simulink model "ASDrf_Governor"  (R2016b)
settings: configuration reference "CodeGenConfigSet" (kept outside this file)
values from neighbouring files (symbols this model uses):
  ASDrf_KpFltCurr_C = Calibration.Parameter    [init_ASDrf_Governor.m]    (also in init_ASDrf_Governor_SIL.m = Simulink.Parameter)
  ASDrf_swtLim_C = Calibration.Parameter    [init_ASDrf_Governor.m]    (also in init_ASDrf_Governor_SIL.m = Simulink.Parameter)
  ASDrf_swtSpdGovCor_C = Calibration.Parameter    [init_ASDrf_Governor.m]    (also in init_ASDrf_Governor_SIL.m = Simulink.Parameter)
  ASDrf_trqSteepNeg_C = Calibration.Parameter    [init_ASDrf_Governor.m]    (also in init_ASDrf_Governor_SIL.m = Simulink.Parameter)
  ASDrf_trqSteepPos_C = Calibration.Parameter    [init_ASDrf_Governor.m]    (also in init_ASDrf_Governor_SIL.m = Simulink.Parameter)
  ASDrf_trqThresNeg_C = Calibration.Parameter    [init_ASDrf_Governor.m]    (also in init_ASDrf_Governor_SIL.m = Simulink.Parameter)
  ASDrf_trqThresPos_C = Calibration.Parameter    [init_ASDrf_Governor.m]    (also in init_ASDrf_Governor_SIL.m = Simulink.Parameter)
  TRQ_MAX = fi(1000,Trq_Nm)    [init_ASDrf_Governor.m]    (also in init_ASDrf_Governor_SIL.m)
  TRQ_MIN = fi(-3276,Trq_Nm)    [init_ASDrf_Governor.m]    (also in init_ASDrf_Governor_SIL.m)
libraries: simulink x10, CXLib x4
settings Model: Creator=lenovo  LastModifiedBy=lenovo
settings ConfigSetRef: SourceLocation=Base Workspace

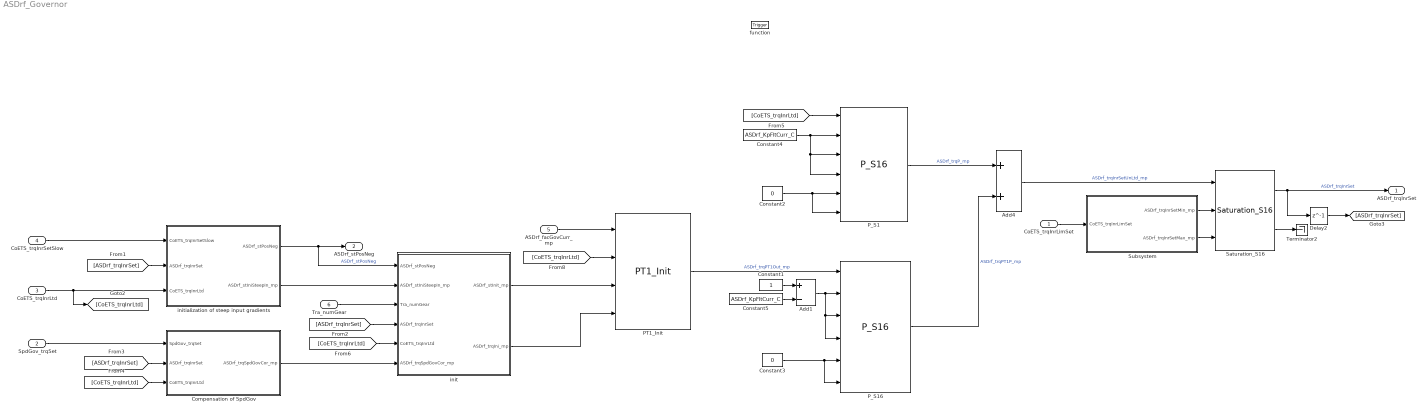
== system ASDrf_Governor ==
  CoETS_trqInrLimSet : Inport  Tag=Nm  Description=Limitation torque without the part of the speed governor  OutMin=-3000  OutMax=3000  OutDataTypeStr=Trq_Nm
  SpdGov_trqSet : Inport  Tag=Nm  Description=Set point torque of SpdGov on the fuel path  Port=2  OutMin=-3000  OutMax=3000  OutDataTypeStr=Trq_Nm
  CoETS_trqInrLtd : Inport  Tag=Nm  Description=inner torque set value after limitation, before AS  Port=3  OutMin=-3000  OutMax=3000  OutDataTypeStr=Trq_Nm
  CoETS_trqInrSetSlow : Inport  Tag=Nm  Description=Filtered inner torque ( positive torque) desired value (standard signal path) generated out of CoPT_trqDesEng  Port=4  OutMin=-3276  OutMax=3276  OutDataTypeStr=Trq_Nm
  ASDrf_facGovCurr_mp : Inport  Description=Active state after priorisation (decimal coded)  Port=5  OutMin=0  OutMax=99.9  OutDataTypeStr=PT_fac
  Tra_numGear : Inport  Description=Current gear information  Port=6  OutMin=-128  OutMax=127  OutDataTypeStr=Tra_num
  function : TriggerPort  TriggerType=function-call  VariantControl=Variant
  Add1 : Sum  Inputs=+-  SaturateOnIntegerOverflow=on  InputSameDT=on
  Add4 : Sum  SaturateOnIntegerOverflow=on  InputSameDT=on
  Compensation of SpdGov : Subsystem
  Constant1 : Constant  RequirementInfo={'other' 'APP_requirements.doc' '@Simulink_requirement_item_25' 'true' '手动开关' '' } %GIDa_04e9130c_3732_46d4_8727_99cf29214165  OutDataTypeStr=Inherit: Inherit via back propagation
  Constant2 : Constant  RequirementInfo={'other' 'APP_requirements.doc' '@Simulink_requirement_item_25' 'true' '手动开关' '' } %GIDa_94a70317_27f7_4a67_bc50_074724e5fa22  Value=0  OutDataTypeStr=Inherit: Inherit via back propagation
  Constant3 : Constant  RequirementInfo={'other' 'APP_requirements.doc' '@Simulink_requirement_item_25' 'true' '手动开关' '' } %GIDa_3fa9db96_13e9_4b77_bcb7_da159fb74a91  Value=0  OutDataTypeStr=Inherit: Inherit via back propagation
  Constant4 : Constant  RequirementInfo={'other' 'APP_requirements.doc' '@Simulink_requirement_item_25' 'true' '手动开关' '' } %GIDa_2e8aa955_92f2_4b22_b779_7d16fefc9cfa  Value=ASDrf_KpFltCurr_C
  Constant5 : Constant  RequirementInfo={'other' 'APP_requirements.doc' '@Simulink_requirement_item_25' 'true' '手动开关' '' } %GIDa_b568d7eb_b45f_4e62_9df6_34760f8c3a7b  Value=ASDrf_KpFltCurr_C
  Delay2 : Delay  DelayLength=1  InitialCondition=0
  PT1_Init : CXLib/PT1_Init
  P_S1 : CXLib/P_S16
  P_S16 : CXLib/P_S16
  Saturation_S16 : CXLib/Saturation_S16
  Subsystem : Subsystem
  Terminator2 : Terminator
  init : Subsystem
  "initialization of steep input gradients " : Subsystem
  ASDrf_trqInrSet : Outport  Tag=Nm  Description=ASD reference filter torque output  OutMin=-3000  OutMax=3000  OutDataTypeStr=Trq_Nm
  ASDrf_stPosNeg : Outport  Description=Positive or negative intervention status  Port=2  OutMin=0  OutMax=1  OutDataTypeStr=boolean
  wires:
  [CoETS_trqInrLtd] -> init/5(CoETS_trqInrLtd)
  Delay2/1 -> [ASDrf_trqInrSet]
  [CoETS_trqInrLtd] -> PT1_Init/2
  Subsystem/2(ASDrf_trqInrSetMax_mp) -> Saturation_S16/3
  Subsystem/1(ASDrf_trqInrSetMin_mp) -> Saturation_S16/2
  CoETS_trqInrLimSet/1 -> Subsystem/1(CoETS_trqInrLimSet)
  "initialization of steep input gradients "/1(ASDrf_stPosNeg) -> ASDrf_stPosNeg/1, init/1(ASDrf_stPosNeg)  "ASDrf_stPosNeg"
  Constant2/1 -> P_S1/6, P_S1/5
  Saturation_S16/2 -> Terminator2/1
  Constant1/1 -> Add1/1
  [ASDrf_trqInrSet] -> Compensation of SpdGov/2(ASDrf_trqInrSet)
  Saturation_S16/1 -> ASDrf_trqInrSet/1, Delay2/1  "ASDrf_trqInrSet"
  P_S16/1 -> Add4/2  "ASDrf_trqPT1P_mp"
  P_S1/1 -> Add4/1  "ASDrf_trqP_mp"
  Constant3/1 -> P_S16/5, P_S16/6
  Add1/1 -> P_S16/2, P_S16/3, P_S16/4
  init/1(ASDrf_stInit_mp) -> PT1_Init/3
  Constant5/1 -> Add1/2
  [ASDrf_trqInrSet] -> init/4(ASDrf_trqInrSet)
  CoETS_trqInrSetSlow/1 -> "initialization of steep input gradients "/1(CoETS_trqInrSetSlow)
  PT1_Init/1 -> P_S16/1  "ASDrf_trqPT1Out_mp"
  [ASDrf_trqInrSet] -> "initialization of steep input gradients "/2(ASDrf_trqInrSet)
  Compensation of SpdGov/1(ASDrf_trqSpdGovCor_mp) -> init/6(ASDrf_trqSpdGovCor_mp)
  init/2(ASDrf_trqIni_mp) -> PT1_Init/4
  Tra_numGear/1 -> init/3(Tra_numGear)
  "initialization of steep input gradients "/2(ASDrf_stIniSteepIn_mp) -> init/2(ASDrf_stIniSteepIn_mp)
  CoETS_trqInrLtd/1 -> [CoETS_trqInrLtd], "initialization of steep input gradients "/3(CoETS_trqInrLtd)
  ASDrf_facGovCurr_mp/1 -> PT1_Init/1
  [CoETS_trqInrLtd] -> Compensation of SpdGov/3(CoETS_trqInrLtd)
  [CoETS_trqInrLtd] -> P_S1/1
  Add4/1 -> Saturation_S16/1  "ASDrf_trqInrSetUnLtd_mp"
  Constant4/1 -> P_S1/2, P_S1/3, P_S1/4
  SpdGov_trqSet/1 -> Compensation of SpdGov/1(SpdGov_trqSet)

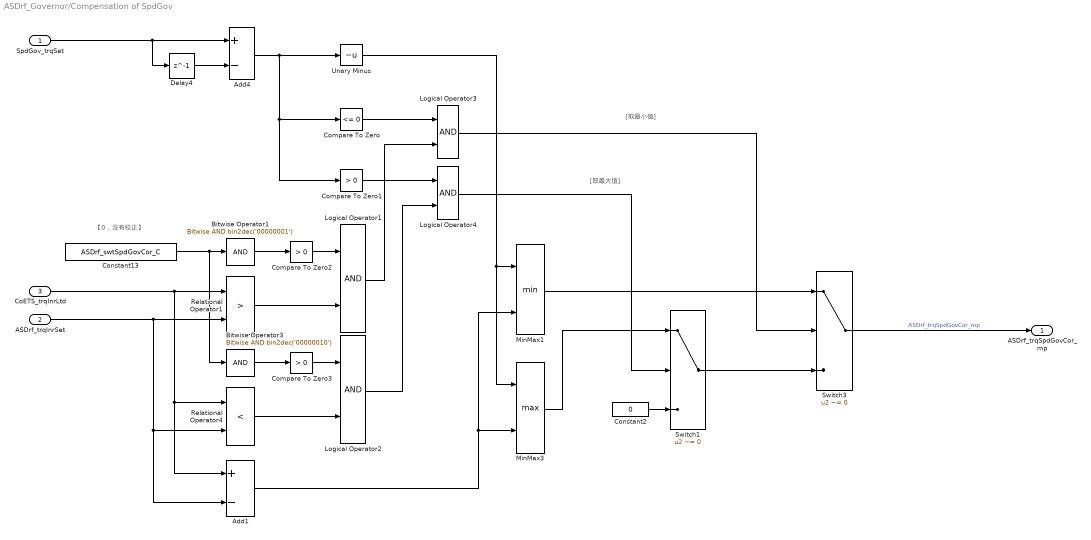
== system ASDrf_Governor/Compensation of SpdGov ==
  note: [取最大值]
  note: [取最小值]
  note: 【0，没有校正】
  SpdGov_trqSet : Inport
  ASDrf_trqInrSet : Inport  Port=2
  CoETS_trqInrLtd : Inport  Port=3
  Add1 : Sum  Inputs=+-  SaturateOnIntegerOverflow=on  InputSameDT=on
  Add4 : Sum  Inputs=+-  SaturateOnIntegerOverflow=on  InputSameDT=on
  Bitwise Operator1 : simulink/Logic and Bit Operations/Bitwise Operator  logicop=AND  UseBitMask=on  BitMask=bin2dec('00000001')  BitMaskRealWorld=Stored Integer
  Bitwise Operator3 : simulink/Logic and Bit Operations/Bitwise Operator  logicop=AND  UseBitMask=on  BitMask=bin2dec('00000010')  BitMaskRealWorld=Stored Integer
  Compare To Zero : simulink/Logic and Bit Operations/Compare To Zero  relop=<=  OutDataTypeStr=boolean
  Compare To Zero1 : simulink/Logic and Bit Operations/Compare To Zero  relop=>  OutDataTypeStr=boolean
  Compare To Zero2 : simulink/Logic and Bit Operations/Compare To Zero  relop=>  OutDataTypeStr=boolean
  Compare To Zero3 : simulink/Logic and Bit Operations/Compare To Zero  relop=>  OutDataTypeStr=boolean
  Constant13 : Constant  RequirementInfo={'other' 'APP_requirements.doc' '@Simulink_requirement_item_25' 'true' '手动开关' '' } %GIDa_336f8dde_0a6f_4504_9b94_889caf0ed8bc  Value=ASDrf_swtSpdGovCor_C  SampleTime=-1
  Constant2 : Constant  RequirementInfo={'other' 'APP_requirements.doc' '@Simulink_requirement_item_25' 'true' '手动开关' '' } %GIDa_e3fc0150_ba4b_4eb3_baf9_a854b361ddb2  Value=0  OutDataTypeStr=Inherit: Inherit via back propagation
  Delay4 : Delay  DelayLength=1  InitialCondition=0
  Logical Operator{1..4} (4 alike) : Logic  OutDataTypeStr=boolean
  MinMax1 : MinMax  Inputs=2  SaturateOnIntegerOverflow=on  InputSameDT=on
  MinMax3 : MinMax  Function=max  Inputs=2  SaturateOnIntegerOverflow=on  InputSameDT=on
  Relational Operator1 : RelationalOperator  Operator=>  OutDataTypeStr=boolean  RndMeth=Simplest  InputSameDT=on
  Relational Operator4 : RelationalOperator  Operator=<  OutDataTypeStr=boolean  RndMeth=Simplest  InputSameDT=on
  Switch1 : Switch  Criteria=u2 ~= 0  SaturateOnIntegerOverflow=on  InputSameDT=on
  Switch3 : Switch  Criteria=u2 ~= 0  SaturateOnIntegerOverflow=on  InputSameDT=on
  Unary Minus : UnaryMinus
  ASDrf_trqSpdGovCor_mp : Outport
  wires:
  Compare To Zero3/1 -> Logical Operator2/1
  Bitwise Operator3/1 -> Compare To Zero3/1
  Compare To Zero2/1 -> Logical Operator1/1
  Constant13/1 -> Bitwise Operator3/1, Bitwise Operator1/1
  SpdGov_trqSet/1 -> Add4/1, Delay4/1
  Switch3/1 -> ASDrf_trqSpdGovCor_mp/1  "ASDrf_trqSpdGovCor_mp"
  Logical Operator1/1 -> Logical Operator3/2
  MinMax1/1 -> Switch3/1
  ASDrf_trqInrSet/1 -> Relational Operator1/2, Relational Operator4/2, Add1/2
  Compare To Zero1/1 -> Logical Operator4/1
  Compare To Zero/1 -> Logical Operator3/1
  CoETS_trqInrLtd/1 -> Relational Operator1/1, Relational Operator4/1, Add1/1
  Relational Operator1/1 -> Logical Operator1/2
  Add4/1 -> Unary Minus/1, Compare To Zero1/1, Compare To Zero/1
  Bitwise Operator1/1 -> Compare To Zero2/1
  MinMax3/1 -> Switch1/1
  Relational Operator4/1 -> Logical Operator2/2
  Logical Operator2/1 -> Logical Operator4/2
  Unary Minus/1 -> MinMax1/1, MinMax3/1
  Logical Operator4/1 -> Switch1/2
  Switch1/1 -> Switch3/3
  Constant2/1 -> Switch1/3
  Delay4/1 -> Add4/2
  Logical Operator3/1 -> Switch3/2
  Add1/1 -> MinMax1/2, MinMax3/2

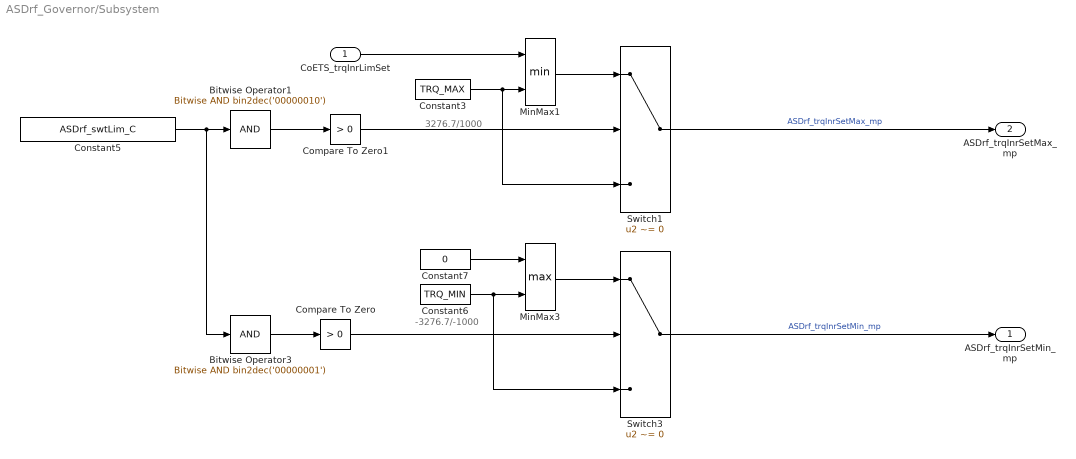
== system ASDrf_Governor/Subsystem ==
  note: 3276.7/1000
  note: -3276.7/-1000
  CoETS_trqInrLimSet : Inport
  Bitwise Operator1 : simulink/Logic and Bit Operations/Bitwise Operator  logicop=AND  UseBitMask=on  BitMask=bin2dec('00000010')  BitMaskRealWorld=Stored Integer
  Bitwise Operator3 : simulink/Logic and Bit Operations/Bitwise Operator  logicop=AND  UseBitMask=on  BitMask=bin2dec('00000001')  BitMaskRealWorld=Stored Integer
  Compare To Zero : simulink/Logic and Bit Operations/Compare To Zero  relop=>  OutDataTypeStr=boolean
  Compare To Zero1 : simulink/Logic and Bit Operations/Compare To Zero  relop=>  OutDataTypeStr=boolean
  Constant3 : Constant  RequirementInfo={'other' 'APP_requirements.doc' '@Simulink_requirement_item_25' 'true' '手动开关' '' } %GIDa_d2a03047_0d49_41bb_a23b_3c875678e112  Value=TRQ_MAX  OutDataTypeStr=Trq_Nm
  Constant5 : Constant  RequirementInfo={'other' 'APP_requirements.doc' '@Simulink_requirement_item_25' 'true' '手动开关' '' } %GIDa_1b8189c9_73f4_417b_b69d_5894943d726c  Value=ASDrf_swtLim_C  SampleTime=-1
  Constant6 : Constant  RequirementInfo={'other' 'APP_requirements.doc' '@Simulink_requirement_item_25' 'true' '手动开关' '' } %GIDa_0c9d292a_2d68_4698_b941_95e69ea20d50  Value=TRQ_MIN  OutDataTypeStr=Trq_Nm
  Constant7 : Constant  RequirementInfo={'other' 'APP_requirements.doc' '@Simulink_requirement_item_25' 'true' '手动开关' '' } %GIDa_fd0df7e2_6efd_409f_b48b_bd2f4b8aa182  Value=0  OutDataTypeStr=Trq_Nm
  MinMax1 : MinMax  Inputs=2  InputSameDT=on
  MinMax3 : MinMax  Function=max  Inputs=2  SaturateOnIntegerOverflow=on  InputSameDT=on
  Switch1 : Switch  Criteria=u2 ~= 0  InputSameDT=on
  Switch3 : Switch  Criteria=u2 ~= 0  InputSameDT=on
  ASDrf_trqInrSetMin_mp : Outport
  ASDrf_trqInrSetMax_mp : Outport  Port=2
  wires:
  Switch1/1 -> ASDrf_trqInrSetMax_mp/1  "ASDrf_trqInrSetMax_mp"
  Constant5/1 -> Bitwise Operator1/1, Bitwise Operator3/1
  MinMax1/1 -> Switch1/1
  CoETS_trqInrLimSet/1 -> MinMax1/1
  Compare To Zero/1 -> Switch3/2
  Constant3/1 -> MinMax1/2, Switch1/3
  Constant6/1 -> MinMax3/2, Switch3/3
  MinMax3/1 -> Switch3/1
  Compare To Zero1/1 -> Switch1/2
  Bitwise Operator3/1 -> Compare To Zero/1
  Bitwise Operator1/1 -> Compare To Zero1/1
  Constant7/1 -> MinMax3/1
  Switch3/1 -> ASDrf_trqInrSetMin_mp/1  "ASDrf_trqInrSetMin_mp"

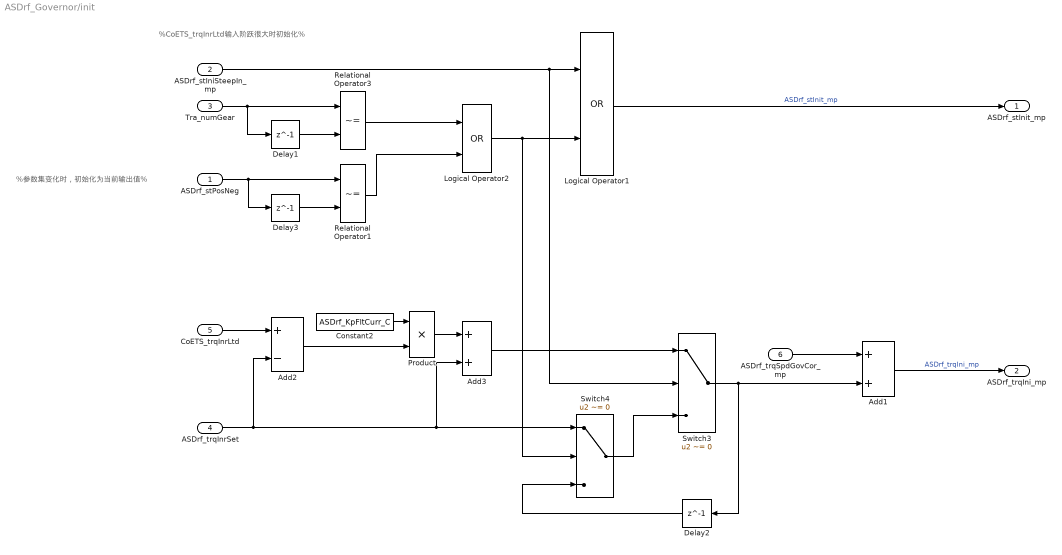
== system ASDrf_Governor/init ==
  note: %CoETS_trqInrLtd输入阶跃很大时初始化%
  note: %参数集变化时，初始化为当前输出值%
  ASDrf_stPosNeg : Inport
  ASDrf_stIniSteepIn_mp : Inport  Port=2
  Tra_numGear : Inport  Port=3
  ASDrf_trqInrSet : Inport  Port=4
  CoETS_trqInrLtd : Inport  Port=5
  ASDrf_trqSpdGovCor_mp : Inport  Port=6
  Add1 : Sum  SaturateOnIntegerOverflow=on  InputSameDT=on
  Add2 : Sum  Inputs=+-  SaturateOnIntegerOverflow=on  InputSameDT=on
  Add3 : Sum  SaturateOnIntegerOverflow=on  InputSameDT=on
  Constant2 : Constant  RequirementInfo={'other' 'APP_requirements.doc' '@Simulink_requirement_item_25' 'true' '手动开关' '' } %GIDa_3e7919d3_3195_4054_bab3_62a9fba2ebc8  Value=ASDrf_KpFltCurr_C
  Delay1 : Delay  DelayLength=1  InitialCondition=0
  Delay2 : Delay  DelayLength=1  InitialCondition=0
  Delay3 : Delay  DelayLength=1  InitialCondition=0
  Logical Operator1 : Logic  Operator=OR  OutDataTypeStr=boolean
  Logical Operator2 : Logic  Operator=OR  OutDataTypeStr=boolean
  Product : Product  OutDataTypeStr=Trq_Nm  SaturateOnIntegerOverflow=on
  Relational Operator1 : RelationalOperator  Operator=~=  OutDataTypeStr=boolean  RndMeth=Simplest  InputSameDT=on
  Relational Operator3 : RelationalOperator  Operator=~=  OutDataTypeStr=boolean  RndMeth=Simplest  InputSameDT=on
  Switch3 : Switch  Criteria=u2 ~= 0  SaturateOnIntegerOverflow=on  InputSameDT=on
  Switch4 : Switch  Criteria=u2 ~= 0  SaturateOnIntegerOverflow=on  InputSameDT=on
  ASDrf_stInit_mp : Outport
  ASDrf_trqIni_mp : Outport  Port=2
  wires:
  Relational Operator1/1 -> Logical Operator2/2
  Relational Operator3/1 -> Logical Operator2/1
  ASDrf_stPosNeg/1 -> Relational Operator1/1, Delay3/1
  Delay3/1 -> Relational Operator1/2
  Tra_numGear/1 -> Relational Operator3/1, Delay1/1
  Delay1/1 -> Relational Operator3/2
  Constant2/1 -> Product/1
  Product/1 -> Add3/1
  Add2/1 -> Product/2
  CoETS_trqInrLtd/1 -> Add2/1
  Add1/1 -> ASDrf_trqIni_mp/1  "ASDrf_trqIni_mp"
  ASDrf_trqInrSet/1 -> Switch4/1, Add3/2, Add2/2
  Add3/1 -> Switch3/1
  Switch4/1 -> Switch3/3
  Delay2/1 -> Switch4/3
  Logical Operator1/1 -> ASDrf_stInit_mp/1  "ASDrf_stInit_mp"
  ASDrf_stIniSteepIn_mp/1 -> Logical Operator1/1, Switch3/2
  Logical Operator2/1 -> Switch4/2, Logical Operator1/2
  ASDrf_trqSpdGovCor_mp/1 -> Add1/1
  Switch3/1 -> Delay2/1, Add1/2

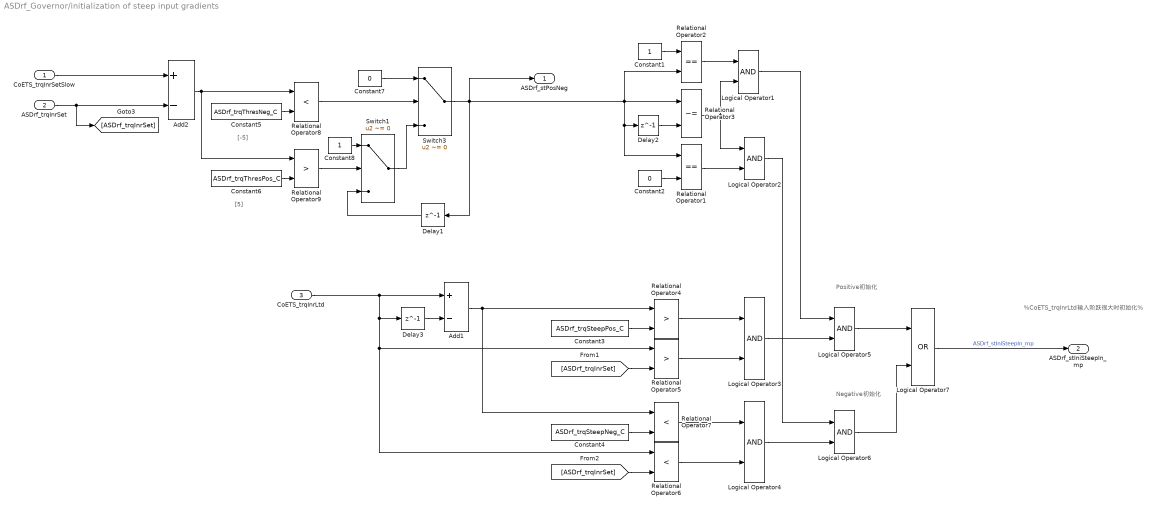
== system ASDrf_Governor/initialization of steep input gradients  ==
  note: Negative初始化
  note: Positive初始化
  note: %CoETS_trqInrLtd输入阶跃很大时初始化%
  note: [-5]
  note: [5]
  CoETS_trqInrSetSlow : Inport
  ASDrf_trqInrSet : Inport  Port=2
  CoETS_trqInrLtd : Inport  Port=3
  Add1 : Sum  Inputs=+-  SaturateOnIntegerOverflow=on  InputSameDT=on
  Add2 : Sum  Inputs=+-  SaturateOnIntegerOverflow=on  InputSameDT=on
  Constant1 : Constant  RequirementInfo={'other' 'APP_requirements.doc' '@Simulink_requirement_item_25' 'true' '手动开关' '' } %GIDa_d8fa8536_6c32_436f_9664_2906f1c65d4b  OutDataTypeStr=boolean
  Constant2 : Constant  RequirementInfo={'other' 'APP_requirements.doc' '@Simulink_requirement_item_25' 'true' '手动开关' '' } %GIDa_5e52f41a_81fb_4bd0_b256_04088d1cba1d  Value=0  OutDataTypeStr=boolean
  Constant3 : Constant  RequirementInfo={'other' 'APP_requirements.doc' '@Simulink_requirement_item_25' 'true' '手动开关' '' } %GIDa_64c9efd0_afa6_48ff_bffd_0814f4788685  Value=ASDrf_trqSteepPos_C  SampleTime=-1
  Constant4 : Constant  RequirementInfo={'other' 'APP_requirements.doc' '@Simulink_requirement_item_25' 'true' '手动开关' '' } %GIDa_ebdd7961_74b8_4757_9274_cbff4b7c0880  Value=ASDrf_trqSteepNeg_C  SampleTime=-1
  Constant5 : Constant  RequirementInfo={'other' 'APP_requirements.doc' '@Simulink_requirement_item_25' 'true' '手动开关' '' } %GIDa_31f54884_b248_4cba_8cec_27d0d87dc9d6  Value=ASDrf_trqThresNeg_C  SampleTime=-1
  Constant6 : Constant  RequirementInfo={'other' 'APP_requirements.doc' '@Simulink_requirement_item_25' 'true' '手动开关' '' } %GIDa_b1d0003b_91c7_4f56_94f5_54d5ded7e3c9  Value=ASDrf_trqThresPos_C  SampleTime=-1
  Constant7 : Constant  RequirementInfo={'other' 'APP_requirements.doc' '@Simulink_requirement_item_25' 'true' '手动开关' '' } %GIDa_d6abebee_b50f_43de_8fb1_71dfa4fbbcc0  Value=0  OutDataTypeStr=boolean
  Constant8 : Constant  RequirementInfo={'other' 'APP_requirements.doc' '@Simulink_requirement_item_25' 'true' '手动开关' '' } %GIDa_7105165d_519c_4442_b02b_7067e87db2a2  OutDataTypeStr=boolean
  Delay1 : Delay  DelayLength=1  InitialCondition=0
  Delay2 : Delay  DelayLength=1  InitialCondition=0
  Delay3 : Delay  DelayLength=1  InitialCondition=0
  Logical Operator{1..6} (6 alike) : Logic  OutDataTypeStr=boolean
  Logical Operator7 : Logic  Operator=OR  OutDataTypeStr=boolean
  Relational Operator1 : RelationalOperator  Operator===  OutDataTypeStr=boolean  RndMeth=Simplest  InputSameDT=on
  Relational Operator2 : RelationalOperator  Operator===  OutDataTypeStr=boolean  RndMeth=Simplest  InputSameDT=on
  Relational Operator3 : RelationalOperator  Operator=~=  OutDataTypeStr=boolean  RndMeth=Simplest  InputSameDT=on
  Relational Operator4 : RelationalOperator  Operator=>  OutDataTypeStr=boolean  RndMeth=Simplest  InputSameDT=on
  Relational Operator5 : RelationalOperator  Operator=>  OutDataTypeStr=boolean  RndMeth=Simplest  InputSameDT=on
  Relational Operator6 : RelationalOperator  Operator=<  OutDataTypeStr=boolean  RndMeth=Simplest  InputSameDT=on
  Relational Operator7 : RelationalOperator  Operator=<  OutDataTypeStr=boolean  RndMeth=Simplest  InputSameDT=on
  Relational Operator8 : RelationalOperator  Operator=<  OutDataTypeStr=boolean  RndMeth=Simplest  InputSameDT=on
  Relational Operator9 : RelationalOperator  Operator=>  OutDataTypeStr=boolean  RndMeth=Simplest  InputSameDT=on
  Switch1 : Switch  Criteria=u2 ~= 0  SaturateOnIntegerOverflow=on  InputSameDT=on
  Switch3 : Switch  Criteria=u2 ~= 0  SaturateOnIntegerOverflow=on  InputSameDT=on
  ASDrf_stPosNeg : Outport
  ASDrf_stIniSteepIn_mp : Outport  Port=2
  wires:
  Delay1/1 -> Switch1/3
  Constant8/1 -> Switch1/1
  Relational Operator9/1 -> Switch1/2
  Switch1/1 -> Switch3/3
  Constant7/1 -> Switch3/1
  Relational Operator8/1 -> Switch3/2
  Constant6/1 -> Relational Operator9/2
  Constant5/1 -> Relational Operator8/2
  Add2/1 -> Relational Operator8/1, Relational Operator9/1
  ASDrf_trqInrSet/1 -> [ASDrf_trqInrSet], Add2/2
  CoETS_trqInrSetSlow/1 -> Add2/1
  Relational Operator5/1 -> Logical Operator3/2
  Relational Operator4/1 -> Logical Operator3/1
  CoETS_trqInrLtd/1 -> Add1/1, Relational Operator6/1, Relational Operator5/1, Delay3/1
  Constant4/1 -> Relational Operator7/2
  Logical Operator4/1 -> Logical Operator6/2
  [ASDrf_trqInrSet] -> Relational Operator6/2
  Relational Operator7/1 -> Logical Operator4/1
  Relational Operator3/1 -> Logical Operator2/1, Logical Operator1/2
  Constant3/1 -> Relational Operator4/2
  Logical Operator6/1 -> Logical Operator7/2
  Constant1/1 -> Relational Operator2/1
  Delay3/1 -> Add1/2
  Logical Operator7/1 -> ASDrf_stIniSteepIn_mp/1  "ASDrf_stIniSteepIn_mp"
  Logical Operator1/1 -> Logical Operator5/1
  Logical Operator3/1 -> Logical Operator5/2
  Add1/1 -> Relational Operator4/1, Relational Operator7/1
  Relational Operator6/1 -> Logical Operator4/2
  Logical Operator5/1 -> Logical Operator7/1
  Logical Operator2/1 -> Logical Operator6/1
  Switch3/1 -> Delay1/1, ASDrf_stPosNeg/1, Relational Operator1/1, Delay2/1, Relational Operator3/1, Relational Operator2/2
  Delay2/1 -> Relational Operator3/2
  Relational Operator1/1 -> Logical Operator2/2
  Constant2/1 -> Relational Operator1/2
  Relational Operator2/1 -> Logical Operator1/1
  [ASDrf_trqInrSet] -> Relational Operator5/2
